simulink model "Washing_Machine_Stateflow"  (R2024b)
settings: Solver=VariableStepAuto  StartTime=0.0  StopTime=inf  RelTol=1e-3
settings Model: Creator=ksamb  LastModifiedBy=suman

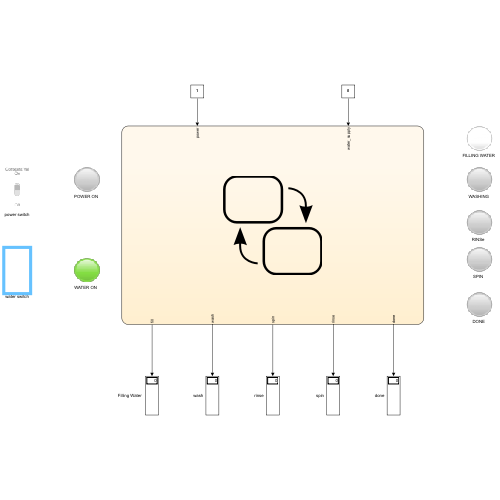
[thumbnail: Simulink's stored preview of the top-level diagram]
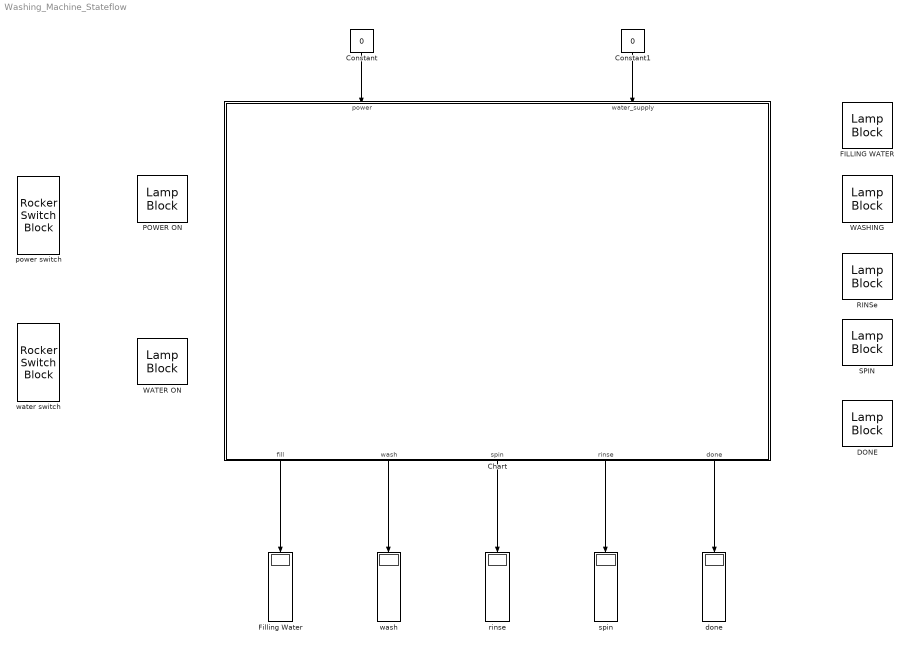
== system Washing_Machine_Stateflow ==
  Chart : Stateflow chart  TreatAsAtomicUnit=on
  Constant : Constant  Value=0
  Constant1 : Constant  Value=0
  DONE : LampBlock  LabelPosition=Hide
  FILLING WATER : LampBlock  LabelPosition=Hide
  "Filling Water " : Display
  POWER ON : LampBlock  LabelPosition=Hide
  "RINSe " : LampBlock  LabelPosition=Hide
  "SPIN " : LampBlock  LabelPosition=Hide
  WASHING : LampBlock  LabelPosition=Hide
  "WATER ON " : LampBlock  LabelPosition=Hide
  done : Display
  power switch : RockerSwitchBlock
      settings: Values={{'Off', 'On'}, [0 1]}
  rinse : Display
  spin : Display
  wash : Display
  water switch : RockerSwitchBlock
      settings: Values={{'Off', 'On'}, [0 1]}
  wires:
  Constant/1 -> Chart/1(power)
  Constant1/1 -> Chart/2(water_supply)
  Chart/1(fill) -> "Filling Water "/1
  Chart/2(wash) -> wash/1
  Chart/3(spin) -> rinse/1
  Chart/5(done) -> done/1
  Chart/4(rinse) -> spin/1

== stateflow chart Washing_Machine_Stateflow/Chart ==
  state power_on
  state water
  state FILL
    entry:fill =1;
  state WASH
    entry:
    fill=0,wash=1;
  state RINSE
    entry:
    wash=0,rinse=1;
  state SPIN
    entry:
    rinse=0,spin=1;
  state DONE
    entry:
    spin=0,done=1;
  (default) -> power_on
  water -> FILL : [water_supply == 1]
  FILL -> WASH : after(10,sec)
  power_on -> water : [power == 1]...
      | {after(3,sec)}
  WASH -> RINSE : after(20,sec)
  RINSE -> SPIN : after(30,sec)
  SPIN -> DONE : after(20,sec)
  data: fill output; wash output; spin output; power input; water_supply input; rinse output; done output
